simulink model "sldemo_househeat"  (R2018a)
settings: Solver=ode45  StartTime=0.0  StopTime=48  FixedStep=1  RelTol=1e-3  AbsTol=1e-6
model workspace (MATLAB code in the model file):
  | % load initial conditions and physical properties from file
  | 
  | sldemo_househeat_data
values from neighbouring files (symbols this model uses):
  c = 1005.4    [sldemo_househeat_data.m]
  M = (len*wid*ht*densAir)    (= 90037.5)    [sldemo_househeat_data.m]
  Mdot = 3538    [sldemo_househeat_data.m]
  Req = RWall    (= 1.74046226678e-08)    [sldemo_househeat_data.m]
  TinIC = 24    [sldemo_househeat_data.m]
Description:
  | Thermal Model of a House
  | 
  | This demo illustrates how you can use Simulink(R) to create the thermal model of
  | a house. This system models the outdoor environment, the thermal
  | characteristics of the house, and the house heating system.
  | 
  | The sldemo_househeat_data.m file initializes data in the model workspace.
  | To make changes, you can edit the model workspace directly or edit the MATLAB(R) file
  | and re-load the model workspace.
  | 
  | To view the model workspace, select View > Model Explorer
  | from the Simulink editor.
  | 
  | Note: Time is given in units of hours
settings Model: ExtModeTrigMode=oneshot  ExtModeArmWhenConnect=off  ExtModeAutoUpdateStatusClock=off  Creator=The MathWorks, Inc.  LastModifiedBy=Coa
settings SolverCC: AutoScaleAbsTol=off
settings DataIOCC: ExternalInput=[]  InitialState=[]  SaveFormat=Array  SaveOutput=off  SaveTime=off  SignalLoggingName=sldemo_househeat_output
settings OptimizationCC: BlockReduction=off  BooleanDataType=off  ExpressionDepthLimit=2147483647  InitFltsAndDblsToZero=on  LifeSpan=inf  BufferReusableBoundary=off
settings DebuggingCC: SaveWithParameterizedLinksMsg=none  UnderspecifiedInitializationDetection=Classic  MergeDetectMultiDrivingBlocksExec=none  SignalResolutionControl=TryResolveAllWithWarning  MultiTaskDSMMsg=warning  MultiTaskCondExecSysMsg=none  IntegerOverflowMsg=none  FcnCallInpInsideContextMsg=warning  BusObjectLabelMismatch=none  StateNameClashWarn=warning  SFUnexpectedBacktrackingDiag=warning  SFNoUnconditionalDefaultTransitionDiag=warning  SFExecutionAtInitializationDiag=none  IntegerSaturationMsg=none
settings HardwareCC: ProdBitPerPointer=32  ProdBitPerSizeT=32  ProdBitPerPtrDiffT=32  ProdLargestAtomicFloat=None  ProdIntDivRoundTo=Undefined  ProdEndianess=Unspecified  ProdWordSize=32  ProdHWDeviceType=32-bit Generic  TargetUnknown=on
settings ModelReferenceCC: PropagateSignalLabelsOutOfModel=off
settings RTWCC: Description=Generic Real-Time Target
settings CodeAppCC: StateflowObjectComments=on
settings GRTTargetCC: TargetFcnLib=ansi_tfl_tmw.mat  TargetLangStandard=C89/C90 (ANSI)  GeneratePreprocessorConditionals=Disable all  CombineOutputUpdateFcns=off  GRTInterface=on
settings ConfigComp: CovMetricSettings=dw  CovHtmlReporting=on  CovSaveCumulativeToWorkspaceVar=on  CovSaveSingleToWorkspaceVar=on  CovExternalEMLEnable=off

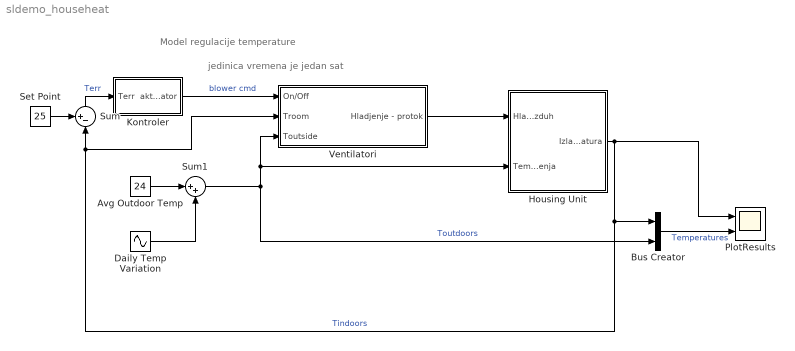
== system sldemo_househeat ==
  note: Model regulacije temperature
  note: jedinica vremena je jedan sat
  Avg Outdoor Temp : Constant  Value=24
  Bus Creator : BusCreator  Inputs=2
  Daily Temp Variation : Sin  Amplitude=2  Frequency=2*pi/24  SampleTime=0
  Housing Unit : Subsystem
  Kontroler : Subsystem
  PlotResults : Scope  NumInputPorts=2
  Set Point : Constant  Value=25
  Sum : Sum  Inputs=+-|  SaturateOnIntegerOverflow=on  InputSameDT=on  OutDataTypeStr=Inherit: Same as first input
  Sum1 : Sum  Inputs=|++  SaturateOnIntegerOverflow=on  InputSameDT=on  OutDataTypeStr=Inherit: Same as first input
  Ventilatori : Subsystem
  wires:
  Kontroler/1(aktivator) -> Ventilatori/1(On/Off)  "blower cmd"
  Sum/1 -> Kontroler/1(Terr)  "Terr"
  Daily Temp Variation/1 -> Sum1/2
  Sum1/1 -> Bus Creator/2, Ventilatori/3(Toutside), Housing Unit/2(Temperatura okruženja)  "Toutdoors"
  Avg Outdoor Temp/1 -> Sum1/1
  Housing Unit/1(Izlazna temperatura) -> Ventilatori/2(Troom), Sum/2, Bus Creator/1, PlotResults/1  "Tindoors"
  Ventilatori/1(Hladjenje - protok) -> Housing Unit/1(Hladan vazduh)
  Bus Creator/1 -> PlotResults/2  "Temperatures"
  Set Point/1 -> Sum/1

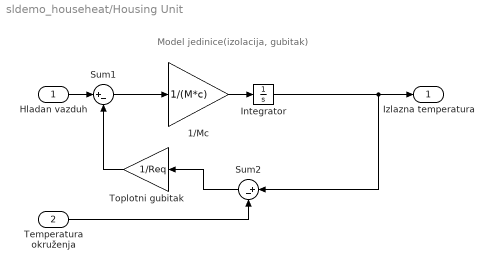
== system sldemo_househeat/Housing Unit ==
  note: Model jedinice(izolacija, gubitak)
  Hladan vazduh : Inport
  Temperatura okruženja : Inport  Port=2
  1/Mc : Gain  Gain=1/(M*c)  SaturateOnIntegerOverflow=on  OutDataTypeStr=Inherit: Same as input  ParamDataTypeStr=Inherit: Same as input
  Integrator : Integrator  InitialCondition=TinIC
  Sum1 : Sum  Inputs=|+-  SaturateOnIntegerOverflow=on  InputSameDT=on  OutDataTypeStr=Inherit: Same as first input
  Sum2 : Sum  Inputs=|+-  SaturateOnIntegerOverflow=on  InputSameDT=on  OutDataTypeStr=Inherit: Same as first input
  Toplotni gubitak : Gain  Gain=1/Req  SaturateOnIntegerOverflow=on  OutDataTypeStr=Inherit: Same as input  ParamDataTypeStr=Inherit: Same as input
  Izlazna temperatura : Outport  InitialOutput=0
  wires:
  Sum1/1 -> 1/Mc/1
  Sum2/1 -> Toplotni gubitak/1
  1/Mc/1 -> Integrator/1
  Integrator/1 -> Sum2/1, Izlazna temperatura/1
  Toplotni gubitak/1 -> Sum1/2
  Hladan vazduh/1 -> Sum1/1
  Temperatura okruženja/1 -> Sum2/2

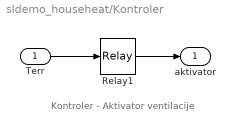
== system sldemo_househeat/Kontroler ==
  note: Kontroler - Aktivator ventilacije
  Terr : Inport
  Relay1 : Relay  OnSwitchValue=5*(5/9)  OffSwitchValue=-5*(5/9)
  aktivator : Outport  InitialOutput=0
  wires:
  Terr/1 -> Relay1/1
  Relay1/1 -> aktivator/1

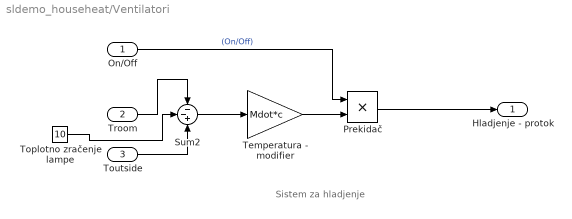
== system sldemo_househeat/Ventilatori ==
  note: Sistem za hladjenje
  On/Off : Inport
  Troom : Inport  Port=2
  Toutside : Inport  Port=3
  Prekidač : Product  RndMeth=Zero
  Sum2 : Sum  Inputs=--+
  Temperatura - modifier : Gain  Gain=Mdot*c
  Toplotno zračenje lampe : Constant  Value=10
  Hladjenje - protok : Outport
  wires:
  Sum2/1 -> Temperatura - modifier/1
  On/Off/1 -> Prekidač/1  "(On/Off)"
  Temperatura - modifier/1 -> Prekidač/2
  Prekidač/1 -> Hladjenje - protok/1
  Troom/1 -> Sum2/1
  Toutside/1 -> Sum2/3
  Toplotno zračenje lampe/1 -> Sum2/2
